simulink library "lib_sensors"  (R2026a)
settings: Solver=VariableStepAuto
undefined symbols (not defined in the file or in its folder): acc_param, lpot_param, random_seed
libraries: simulink x2
settings Model: Creator=alessandro-nardin  LastModifiedBy=alessandro-nardin

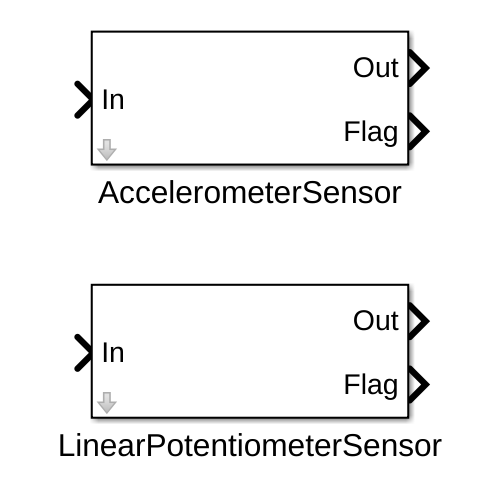
[thumbnail: Simulink's stored preview of the top-level diagram]
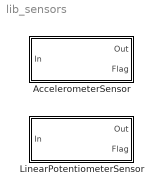
== system lib_sensors ==
  AccelerometerSensor : Subsystem  mask{out_sample_t=0}
      mask prompts: out_sample_t "Sample Time of Output (flag generation)"
  LinearPotentiometerSensor : Subsystem  mask{out_sample_t=0}
      mask prompts: out_sample_t "Sample Time of output (flag generation)"

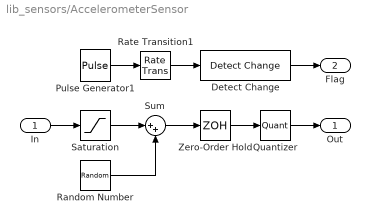
== system lib_sensors/AccelerometerSensor ==
  In : Inport
  Detect Change : simulink/Logic and Bit Operations/Detect Change  vinit=0  OutDataTypeStr=uint8
  Pulse Generator1 : DiscretePulseGenerator  SampleTime=acc_param.sample_t
  Quantizer : Quantizer  QuantizationInterval=acc_param.q_step
  Random Number : RandomNumber  Variance=acc_param.noise_var  Seed=random_seed  SampleTime=acc_param.sample_t
  Rate Transition1 : RateTransition  Deterministic=off  OutPortSampleTime=out_sample_t
  Saturation : Saturate  UpperLimit=acc_param.max_acc  LowerLimit=acc_param.min_acc
  Sum : Sum  Inputs=|++
  Zero-Order Hold : ZeroOrderHold  SampleTime=acc_param.sample_t
  Out : Outport
  Flag : Outport  Port=2
  wires:
  Random Number/1 -> Sum/2
  Quantizer/1 -> Out/1
  In/1 -> Saturation/1
  Sum/1 -> Zero-Order Hold/1
  Zero-Order Hold/1 -> Quantizer/1
  Detect Change/1 -> Flag/1
  Pulse Generator1/1 -> Rate Transition1/1
  Rate Transition1/1 -> Detect Change/1
  Saturation/1 -> Sum/1

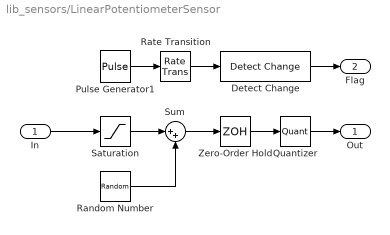
== system lib_sensors/LinearPotentiometerSensor ==
  In : Inport
  Detect Change : simulink/Logic and Bit Operations/Detect Change  vinit=0  OutDataTypeStr=uint8
  Pulse Generator1 : DiscretePulseGenerator  SampleTime=lpot_param.sample_t
  Quantizer : Quantizer  QuantizationInterval=lpot_param.q_step  LinearizeAsGain=off
  Random Number : RandomNumber  Variance=lpot_param.noise_var  Seed=random_seed+1  SampleTime=lpot_param.sample_t
  Rate Transition : RateTransition  Deterministic=off  OutPortSampleTime=out_sample_t
  Saturation : Saturate  UpperLimit=lpot_param.max_d  LowerLimit=lpot_param.min_d
  Sum : Sum  Inputs=|++
  Zero-Order Hold : ZeroOrderHold  SampleTime=lpot_param.sample_t
  Out : Outport
  Flag : Outport  Port=2
  wires:
  In/1 -> Saturation/1
  Random Number/1 -> Sum/2
  Saturation/1 -> Sum/1
  Sum/1 -> Zero-Order Hold/1
  Quantizer/1 -> Out/1
  Detect Change/1 -> Flag/1
  Rate Transition/1 -> Detect Change/1
  Pulse Generator1/1 -> Rate Transition/1
  Zero-Order Hold/1 -> Quantizer/1
